simulink model "CDR_Basic_lib"  (R2012b)
settings: Solver=ode45  StartTime=0.0  StopTime=10.0  RelTol=1e-3
values from neighbouring files (symbols this model uses):
  Ts = 1/fbit/OSR    (= 0.01)    [init_pr_bb_cdr.m]
undefined symbols (not defined in the file): Fosc, Int_Divider, Tsymbol, VDD
libraries: simulink_extras x124, simulink x3
(part 2 of 2)

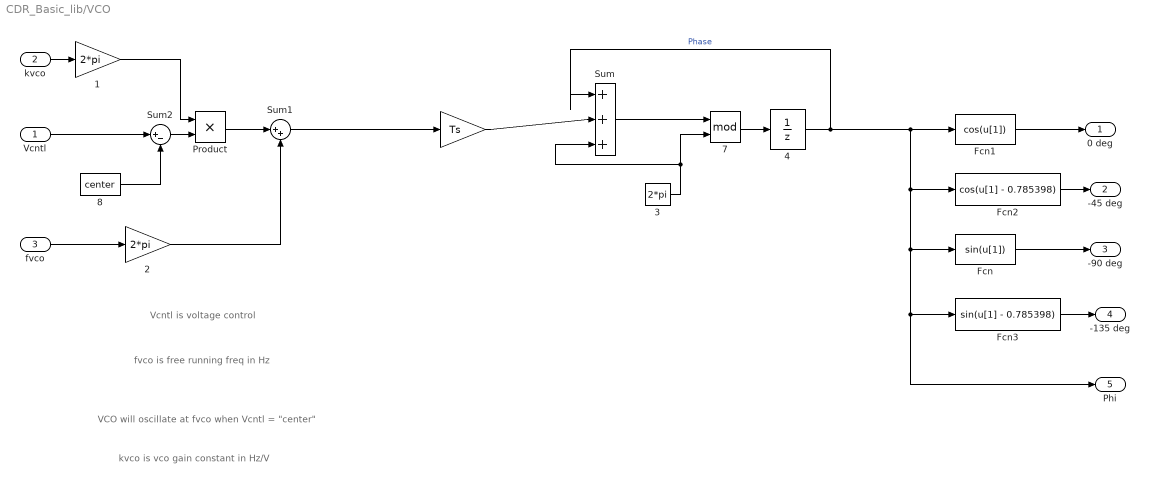
== system CDR_Basic_lib/VCO ==
  note: fvco is free running
      | freq in Hz
  note: kvco is vco gain
      | constant in Hz/V
  note: Vcntl is voltage control
  note: VCO will oscillate at fvco
      | when Vcntl = "center"
  Vcntl : Inport
  kvco : Inport  Port=2
  fvco : Inport  Port=3
  " " : Gain  Gain=Ts  SaturateOnIntegerOverflow=on  OutDataTypeStr=Inherit: Same as input  ParamDataTypeStr=Inherit: Same as input
  " 1" : Gain  Gain=2*pi  SaturateOnIntegerOverflow=on  OutDataTypeStr=Inherit: Same as input  ParamDataTypeStr=Inherit: Same as input
  " 2" : Gain  Gain=2*pi  SaturateOnIntegerOverflow=on  OutDataTypeStr=Inherit: Same as input  ParamDataTypeStr=Inherit: Same as input
  3 : Constant  Value=2*pi
  4 : UnitDelay  InitialCondition=ph_init  SampleTime=Ts
  7 : Math  Operator=mod  SaturateOnIntegerOverflow=on
  8 : Constant  Value=center
  Fcn : Fcn  SampleTime=Ts
  Fcn1 : Fcn  Expr=cos(u[1])  SampleTime=Ts
  Fcn2 : Fcn  Expr=cos(u[1] - 0.785398)  SampleTime=Ts
  Fcn3 : Fcn  Expr=sin(u[1] - 0.785398)  SampleTime=Ts
  Product : Product  SaturateOnIntegerOverflow=on  InputSameDT=on  OutDataTypeStr=Inherit: Same as first input
  Sum : Sum  Inputs=|+++  SaturateOnIntegerOverflow=on  InputSameDT=on  OutDataTypeStr=Inherit: Same as first input
  Sum1 : Sum  Inputs=|++  SaturateOnIntegerOverflow=on  InputSameDT=on  OutDataTypeStr=Inherit: Same as first input
  Sum2 : Sum  Inputs=|+-  SaturateOnIntegerOverflow=on  InputSameDT=on  OutDataTypeStr=Inherit: Same as first input
  0 deg : Outport
  -45 deg : Outport  Port=2
  -90 deg : Outport  Port=3
  -135 deg : Outport  Port=4
  Phi : Outport  Port=5
  wires:
  Fcn3/1 -> -135 deg/1
  Fcn2/1 -> -45 deg/1
  3/1 -> Sum/3, 7/2
  Fcn1/1 -> 0 deg/1
  Fcn/1 -> -90 deg/1
  Product/1 -> Sum1/1
  " 1"/1 -> Product/1
  kvco/1 -> " 1"/1
  fvco/1 -> " 2"/1
  " 2"/1 -> Sum1/2
  Sum2/1 -> Product/2
  Vcntl/1 -> Sum2/1
  8/1 -> Sum2/2
  " "/1 -> Sum/2
  Sum/1 -> 7/1
  Sum1/1 -> " "/1
  7/1 -> 4/1
  4/1 -> Fcn1/1, Fcn2/1, Fcn/1, Phi/1, Fcn3/1, Sum/1  "Phase"

== system CDR_Basic_lib/VCO Phase ==
  note: VCO will oscillate at fvco
      | when Vcntl = "center"
  note: Vcntl is voltage control
  note: kvco is vco gain
      | constant in Hz/V
  note: fvco is free running
      | freq in Hz
  Vcntl : Inport
  kvco : Inport  Port=2
  fvco : Inport  Port=3
  " " : Gain  Gain=Ts  SaturateOnIntegerOverflow=on  OutDataTypeStr=Inherit: Same as input  ParamDataTypeStr=Inherit: Same as input
  " 1" : Gain  Gain=2*pi  SaturateOnIntegerOverflow=on  OutDataTypeStr=Inherit: Same as input  ParamDataTypeStr=Inherit: Same as input
  " 2" : Gain  Gain=2*pi  SaturateOnIntegerOverflow=on  OutDataTypeStr=Inherit: Same as input  ParamDataTypeStr=Inherit: Same as input
  3 : Constant  Value=2*pi
  4 : UnitDelay  InitialCondition=ph_init  SampleTime=Ts
  7 : Math  Operator=mod  SaturateOnIntegerOverflow=on
  8 : Constant  Value=center
  Product : Product  SaturateOnIntegerOverflow=on  InputSameDT=on  OutDataTypeStr=Inherit: Same as first input
  Sum : Sum  Inputs=|+++  SaturateOnIntegerOverflow=on  InputSameDT=on  OutDataTypeStr=Inherit: Same as first input
  Sum1 : Sum  Inputs=|++  SaturateOnIntegerOverflow=on  InputSameDT=on  OutDataTypeStr=Inherit: Same as first input
  Sum2 : Sum  Inputs=|+-  SaturateOnIntegerOverflow=on  InputSameDT=on  OutDataTypeStr=Inherit: Same as first input
  Phi : Outport
  wires:
  4/1 -> Sum/1, Phi/1  "Phase"
  7/1 -> 4/1
  Sum1/1 -> " "/1
  Sum/1 -> 7/1
  " "/1 -> Sum/2
  8/1 -> Sum2/2
  Vcntl/1 -> Sum2/1
  Sum2/1 -> Product/2
  " 2"/1 -> Sum1/2
  fvco/1 -> " 2"/1
  kvco/1 -> " 1"/1
  " 1"/1 -> Product/1
  Product/1 -> Sum1/1
  3/1 -> 7/2, Sum/3

== system CDR_Basic_lib/div ==
  In : Inport
  7 : Math  Operator=mod  SaturateOnIntegerOverflow=on
  FIXED : Constant
  Logical Operator : Logic  AllPortsSameDT=off  OutDataTypeStr=boolean
  Sum5 : Sum  Inputs=|++  OutDataTypeStr=double
  Unit Delay : UnitDelay  SampleTime=-1
  cmp : simulink/Logic and Bit Operations/Compare To Constant  relop=<  const=Div_Rat  OutDataTypeStr=boolean  ZeroCross=off
  cmp1 : simulink/Logic and Bit Operations/Compare To Constant  relop=>=  const=round(Div_Rat/2)  OutDataTypeStr=boolean  ZeroCross=off
  cmp2 : simulink/Logic and Bit Operations/Compare To Constant  relop=<  const=round(1.5*Div_Rat)  OutDataTypeStr=boolean  ZeroCross=off
  div : Constant  Value=2*Div_Rat
  register : Subsystem
  OutR : Outport  InitialOutput=0
  OutQ : Outport  Port=2  InitialOutput=0
  wires:
  In/1 -> register/Trigger
  register/1(Out1) -> Unit Delay/1, cmp1/1, cmp2/1, cmp/1
  FIXED/1 -> Sum5/1
  7/1 -> register/1(In1)
  Sum5/1 -> 7/1
  div/1 -> 7/2
  cmp/1 -> OutR/1
  Unit Delay/1 -> Sum5/2
  cmp1/1 -> Logical Operator/1
  cmp2/1 -> Logical Operator/2
  Logical Operator/1 -> OutQ/1

== system CDR_Basic_lib/1//2-Rate BB PD/DFF1 ==
  D : Inport  LatchByDelayingOutsideSignal=on
  Trigger : TriggerPort
  High Value : Constant  Value=DataHigh
  Low Value : Constant  Value=DataLow
  Switch : Switch  Threshold=FF_Threshold
  Q : Outport
  wires:
  Low Value/1 -> Switch/3
  High Value/1 -> Switch/1
  D/1 -> Switch/2
  Switch/1 -> Q/1

== system CDR_Basic_lib/1//2-Rate BB PD/DFF2 ==
  D : Inport  LatchByDelayingOutsideSignal=on
  Trigger : TriggerPort
  High Value : Constant  Value=DataHigh
  Low Value : Constant  Value=DataLow
  Switch : Switch  Threshold=FF_Threshold
  Q : Outport
  wires:
  Low Value/1 -> Switch/3
  High Value/1 -> Switch/1
  D/1 -> Switch/2
  Switch/1 -> Q/1

== system CDR_Basic_lib/1//2-Rate BB PD/DFF3 ==
  D : Inport  LatchByDelayingOutsideSignal=on
  Trigger : TriggerPort
  High Value : Constant  Value=DataHigh
  Low Value : Constant  Value=DataLow
  Switch : Switch  Threshold=FF_Threshold
  Q : Outport
  wires:
  Low Value/1 -> Switch/3
  High Value/1 -> Switch/1
  D/1 -> Switch/2
  Switch/1 -> Q/1

== system CDR_Basic_lib/1//2-Rate BB PD/DFF4 ==
  D : Inport  LatchByDelayingOutsideSignal=on
  Trigger : TriggerPort
  High Value : Constant  Value=DataHigh
  Low Value : Constant  Value=DataLow
  Switch : Switch  Threshold=FF_Threshold
  Q : Outport
  wires:
  Switch/1 -> Q/1
  D/1 -> Switch/2
  High Value/1 -> Switch/1
  Low Value/1 -> Switch/3

== system CDR_Basic_lib/1//2-Rate BB PD/DFF5 ==
  D : Inport  LatchByDelayingOutsideSignal=on
  Trigger : TriggerPort
  High Value : Constant  Value=DataHigh
  Low Value : Constant  Value=DataLow
  Switch : Switch  Threshold=FF_Threshold
  Q : Outport
  wires:
  Low Value/1 -> Switch/3
  High Value/1 -> Switch/1
  D/1 -> Switch/2
  Switch/1 -> Q/1

== system CDR_Basic_lib/1//2-Rate BB PD/DFF6 ==
  D : Inport  LatchByDelayingOutsideSignal=on
  Trigger : TriggerPort
  High Value : Constant  Value=DataHigh
  Low Value : Constant  Value=DataLow
  Switch : Switch  Threshold=FF_Threshold
  Q : Outport
  wires:
  Low Value/1 -> Switch/3
  High Value/1 -> Switch/1
  D/1 -> Switch/2
  Switch/1 -> Q/1

== system CDR_Basic_lib/1//2-Rate BB PD/DFF7 ==
  D : Inport  LatchByDelayingOutsideSignal=on
  Trigger : TriggerPort
  High Value : Constant  Value=DataHigh
  Low Value : Constant  Value=DataLow
  Switch : Switch  Threshold=FF_Threshold
  Q : Outport
  wires:
  Switch/1 -> Q/1
  D/1 -> Switch/2
  High Value/1 -> Switch/1
  Low Value/1 -> Switch/3

== system CDR_Basic_lib/1//2-Rate BB PD/DFF8 ==
  D : Inport  LatchByDelayingOutsideSignal=on
  Trigger : TriggerPort
  High Value : Constant  Value=DataHigh
  Low Value : Constant  Value=DataLow
  Switch : Switch  Threshold=FF_Threshold
  Q : Outport
  wires:
  Low Value/1 -> Switch/3
  High Value/1 -> Switch/1
  D/1 -> Switch/2
  Switch/1 -> Q/1

== system CDR_Basic_lib/:Linear PD/DLatch ==
  D : Inport
  Clk : Inport  Port=2
  Constant : Constant  Value=L_Threshold
  D Latch : simulink_extras/Flip Flops/D Latch
  Data Type Conversion1 : DataTypeConversion  OutDataTypeStr=boolean
  Data Type Conversion2 : DataTypeConversion  OutDataTypeStr=double
  Data Type Conversion3 : DataTypeConversion  OutDataTypeStr=double
  Gain : Gain  Gain=DataHigh
  Gain1 : Gain  Gain=DataHigh
  Relational Operator : RelationalOperator  OutDataTypeStr=boolean
  Q : Outport
  wires:
  Constant/1 -> Relational Operator/2
  Relational Operator/1 -> D Latch/1
  Data Type Conversion3/1 -> Gain1/1
  Gain/1 -> Q/1
  Data Type Conversion2/1 -> Gain/1
  D Latch/2 -> Data Type Conversion3/1
  D Latch/1 -> Data Type Conversion2/1
  Data Type Conversion1/1 -> D Latch/2
  Clk/1 -> Data Type Conversion1/1
  D/1 -> Relational Operator/1

== system CDR_Basic_lib/:Linear PD/DLatch1 ==
  D : Inport
  Clk : Inport  Port=2
  Constant : Constant  Value=L_Threshold
  D Latch : simulink_extras/Flip Flops/D Latch
  Data Type Conversion1 : DataTypeConversion  OutDataTypeStr=boolean
  Data Type Conversion2 : DataTypeConversion  OutDataTypeStr=double
  Data Type Conversion3 : DataTypeConversion  OutDataTypeStr=double
  Gain : Gain  Gain=DataHigh
  Gain1 : Gain  Gain=DataHigh
  Relational Operator : RelationalOperator  OutDataTypeStr=boolean
  Q : Outport
  wires:
  Constant/1 -> Relational Operator/2
  Relational Operator/1 -> D Latch/1
  Data Type Conversion3/1 -> Gain1/1
  Gain/1 -> Q/1
  Data Type Conversion2/1 -> Gain/1
  D Latch/2 -> Data Type Conversion3/1
  D Latch/1 -> Data Type Conversion2/1
  Data Type Conversion1/1 -> D Latch/2
  Clk/1 -> Data Type Conversion1/1
  D/1 -> Relational Operator/1

== system CDR_Basic_lib/:Linear PD/DLatch2 ==
  D : Inport
  Clk : Inport  Port=2
  Constant : Constant  Value=L_Threshold
  D Latch : simulink_extras/Flip Flops/D Latch
  Data Type Conversion1 : DataTypeConversion  OutDataTypeStr=boolean
  Data Type Conversion2 : DataTypeConversion  OutDataTypeStr=double
  Data Type Conversion3 : DataTypeConversion  OutDataTypeStr=double
  Gain : Gain  Gain=DataHigh
  Gain1 : Gain  Gain=DataHigh
  Relational Operator : RelationalOperator  OutDataTypeStr=boolean
  Q : Outport
  wires:
  Constant/1 -> Relational Operator/2
  Relational Operator/1 -> D Latch/1
  Data Type Conversion3/1 -> Gain1/1
  Gain/1 -> Q/1
  Data Type Conversion2/1 -> Gain/1
  D Latch/2 -> Data Type Conversion3/1
  D Latch/1 -> Data Type Conversion2/1
  Data Type Conversion1/1 -> D Latch/2
  Clk/1 -> Data Type Conversion1/1
  D/1 -> Relational Operator/1

== system CDR_Basic_lib/:Linear PD/DLatch3 ==
  D : Inport
  Clk : Inport  Port=2
  Constant : Constant  Value=L_Threshold
  D Latch : simulink_extras/Flip Flops/D Latch
  Data Type Conversion1 : DataTypeConversion  OutDataTypeStr=boolean
  Data Type Conversion2 : DataTypeConversion  OutDataTypeStr=double
  Data Type Conversion3 : DataTypeConversion  OutDataTypeStr=double
  Gain : Gain  Gain=DataHigh
  Gain1 : Gain  Gain=DataHigh
  Relational Operator : RelationalOperator  OutDataTypeStr=boolean
  Q : Outport
  wires:
  Constant/1 -> Relational Operator/2
  Relational Operator/1 -> D Latch/1
  Data Type Conversion3/1 -> Gain1/1
  Gain/1 -> Q/1
  Data Type Conversion2/1 -> Gain/1
  D Latch/2 -> Data Type Conversion3/1
  D Latch/1 -> Data Type Conversion2/1
  Data Type Conversion1/1 -> D Latch/2
  Clk/1 -> Data Type Conversion1/1
  D/1 -> Relational Operator/1

== system CDR_Basic_lib/InterfacePDBB/DFF2 ==
  D : Inport  LatchByDelayingOutsideSignal=on
  Trigger : TriggerPort
  High Value : Constant  Value=DataHigh
  Low Value : Constant  Value=DataLow
  Switch : Switch  Threshold=FF_Threshold
  Q : Outport
  wires:
  Switch/1 -> Q/1
  D/1 -> Switch/2
  High Value/1 -> Switch/1
  Low Value/1 -> Switch/3

== system CDR_Basic_lib/InterfacePDBB/DFF3 ==
  D : Inport  LatchByDelayingOutsideSignal=on
  Trigger : TriggerPort
  High Value : Constant  Value=DataHigh
  Low Value : Constant  Value=DataLow
  Switch : Switch  Threshold=FF_Threshold
  Q : Outport
  wires:
  Switch/1 -> Q/1
  D/1 -> Switch/2
  High Value/1 -> Switch/1
  Low Value/1 -> Switch/3

== system CDR_Basic_lib/PDBB/DFF1 ==
  D : Inport  LatchByDelayingOutsideSignal=on
  Trigger : TriggerPort
  High Value : Constant  Value=DataHigh
  Low Value : Constant  Value=DataLow
  Switch : Switch  Threshold=FF_Threshold
  Q : Outport
  wires:
  Switch/1 -> Q/1
  D/1 -> Switch/2
  High Value/1 -> Switch/1
  Low Value/1 -> Switch/3

== system CDR_Basic_lib/PDBB/DFF2 ==
  D : Inport  LatchByDelayingOutsideSignal=on
  Trigger : TriggerPort
  High Value : Constant  Value=DataHigh
  Low Value : Constant  Value=DataLow
  Switch : Switch  Threshold=FF_Threshold
  Q : Outport
  wires:
  Switch/1 -> Q/1
  D/1 -> Switch/2
  High Value/1 -> Switch/1
  Low Value/1 -> Switch/3

== system CDR_Basic_lib/PDBB/DFF3 ==
  D : Inport  LatchByDelayingOutsideSignal=on
  Trigger : TriggerPort
  High Value : Constant  Value=DataHigh
  Low Value : Constant  Value=DataLow
  Switch : Switch  Threshold=FF_Threshold
  Q : Outport
  wires:
  Switch/1 -> Q/1
  D/1 -> Switch/2
  High Value/1 -> Switch/1
  Low Value/1 -> Switch/3

== system CDR_Basic_lib/PDBB/DFF5 ==
  D : Inport  LatchByDelayingOutsideSignal=on
  Trigger : TriggerPort
  High Value : Constant  Value=DataHigh
  Low Value : Constant  Value=DataLow
  Switch : Switch  Threshold=FF_Threshold
  Q : Outport
  wires:
  Switch/1 -> Q/1
  D/1 -> Switch/2
  High Value/1 -> Switch/1
  Low Value/1 -> Switch/3

== system CDR_Basic_lib/div/register ==
  In1 : Inport
  Trigger : TriggerPort  TriggerType=either
  Out1 : Outport
  wires:
  In1/1 -> Out1/1
